simulink model "buck_converter"  (R2020b)
settings: Solver=FixedStepDiscrete  StartTime=0.0  StopTime=1  RelTol=1e-3
undefined symbols (not defined in the file): Acid, Lead
libraries: powerlib x15, powerlib_meascontrol x2, electricdrivelib x1
settings Model: SimulationMode=accelerator  Creator=emin3  LastModifiedBy=emin3
settings DebuggingCC: ArithmeticOperatorsInVariantConditions=warning
settings SFSimCC: CustomCodeUndefinedFunction=UseInterfaceOnly

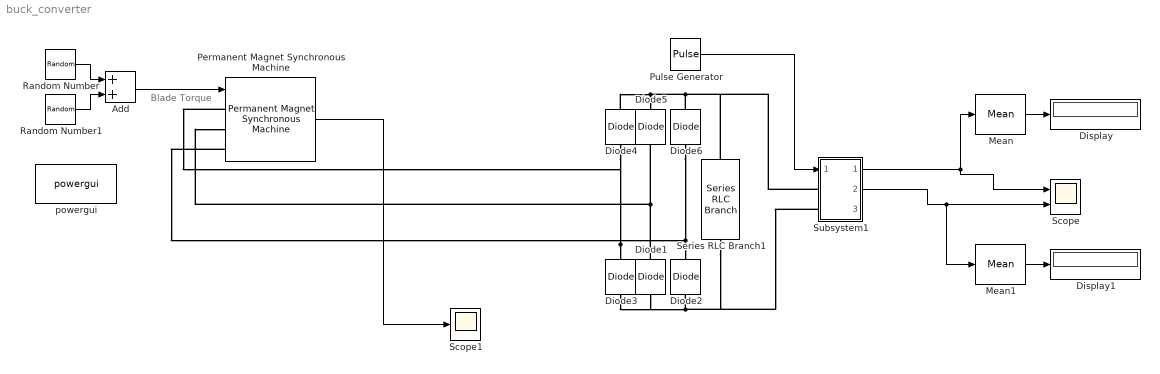
== system buck_converter ==
  note: Blade Torque
  Add : Sum
  Diode{1..6} (6 alike) : powerlib/Power Electronics/Diode  Ron=1e-9  Lon=0  Vf=0.8  IC=0  UseSnubber=0  Rs=1e-6  Cs=250e-9  Measurements=off
  Display : Display
  Display1 : Display
  Mean : powerlib_meascontrol/Measurements/Mean  Freq=60000  Vinit=0  Ts=1e-5
  Mean1 : powerlib_meascontrol/Measurements/Mean  Freq=60000  Vinit=0  Ts=1e-5
  Permanent Magnet Synchronous Machine : powerlib/Machines/Permanent Magnet Synchronous Machine  NbPhases=3  FluxDistribution=Sinusoidal  RotorType=Round  MechanicalLoad=Torque Tm  PresetModel=No  ShowDetailedParameters=on  MeasurementBus=off  Resistance=10.58  Inductance=8.5e-3  dqInductances=[8.5e-3,8.5e-3]  La=0.0167  MachineConstant=Voltage Constant (V_peak L-L / krpm)  Flux=0.60646  VoltageCst=110  TorqueCst=0.90969  Flat=120  Mechanical=[0.00027 0.005024 1 0]  PolePairs=4  InitialConditions=[300,0, 0,0]  InitialConditions5ph=[0 0 0 0 0 0]  RefAngle=90 degrees behind phase A axis (modified Park)  IterativeDiscreteModel=Trapezoidal non iterative  TsBlock=-1  TsPowergui=0
  Pulse Generator : DiscretePulseGenerator  PulseType=Time based  Period=1/6000  PulseWidth=50
  Random Number : RandomNumber  Mean=-1.6  Variance=0.05  SampleTime=1
  Random Number1 : RandomNumber  Variance=0.1  SampleTime=1e-3
  Scope : Scope  NumInputPorts=2
  Scope1 : Scope
  Series RLC Branch1 : powerlib/Elements/Series RLC Branch  LConnTagsString=__new0  RConnTagsString=__new0  BranchType=C  Resistance=20  Inductance=1e-3  SetiL0=off  InitialCurrent=0  Capacitance=1e-6  Setx0=off  InitialVoltage=0  Measurements=None
  Subsystem1 : Subsystem
  powergui : powerlib/powergui  Priority=1  SimulationMode=Discrete  SampleTime=1e-5  frequency=60  Iterations=50  frequencyindice=0  Pbase=100e6  ErrMax=1e-4  UnitsV=kV  UnitsW=MW  buscounter=0  FunctionMessages=off  echomessages=off  EnableUseOfTLC=off  CurrentSourceSwitches=off  DisableSnubberDevices=off  DisableRonSwitches=off  DisableVfSwitches=off  DisplayEquations=off  AutomaticDiscreteSolvers=off  SolverType=Tustin/Backward Euler (TBE)  Interpol=off  ExternalGateDelay=off  methode=off  Ts=100  x0status=blocks  SPID=on  SwTol=0  HookPort=off  NonlinearTolerance=1e-4  nMaxIteration=100  ContinueOnMaxIteration=off  RestoreLinks=warning  ResistiveCurrentMeasurement=off  Frange=[0:2:500]  Ylog=off  Xlog=on  ShowGrid=off  save=off  variable=ZData  structure=0  ZoomFFT=off  StartTime=0.0  cycles=1  DisplayStyle=1  fundamental=60  FreqAxis=off  MaxFrequency=1000  frequencyindicesteady=1  RmsSteady=1  display=off
  wires:
  Random Number/1 -> Add/1
  Add/1 -> Permanent Magnet Synchronous Machine/1
  Random Number1/1 -> Add/2
  Subsystem1/1(Out1) -> Scope/1, Mean/1
  Pulse Generator/1 -> Subsystem1/1(In1)
  Mean/1 -> Display/1
  Mean1/1 -> Display1/1
  Subsystem1/2(Out2) -> Mean1/1, Scope/2
  Permanent Magnet Synchronous Machine/1 -> Scope1/1
  connections:
  Diode6/LConn1 -- Permanent Magnet Synchronous Machine/LConn3 -- Diode2/RConn1
  Diode2/LConn1 -- Diode3/LConn1 -- Diode1/LConn1 -- Subsystem1/LConn2 -- Series RLC Branch1/RConn1
  Diode5/RConn1 -- Diode4/RConn1 -- Subsystem1/LConn1 -- Series RLC Branch1/LConn1 -- Diode6/RConn1
  Diode3/RConn1 -- Permanent Magnet Synchronous Machine/LConn1 -- Diode4/LConn1
  Diode1/RConn1 -- Permanent Magnet Synchronous Machine/LConn2 -- Diode5/LConn1

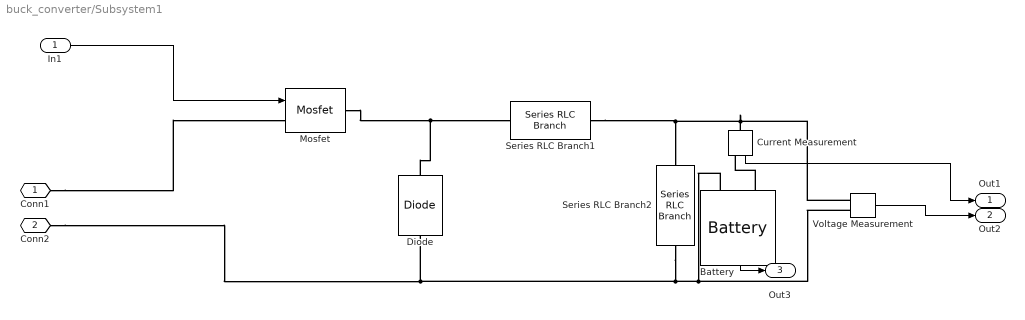
== system buck_converter/Subsystem1 ==
  In1 : Inport
  Battery : electricdrivelib/Extra Sources/Battery  BatType=Lead-Acid  ShowTempParam=off  ThermalPreset=no  ShowAgeParam=off  NomV=24  NomQ=5.4  SOC=50  Batt_Tr=30  PresetModel=on  MaxQ=5.625  MinV=18  FullV=26.1316  Dis_rate=1.08  R=0.044444  Normal_OP=1.6755  expZone="[24.4342        0.018]"  current=[6.5 13 32.5]  Units=Time  Tci=20  NomT=20  T2=-30  MaxQ2=4.8  FullV2=7.1  Normal_OP2=5.655  expZone2="[6.58           1]"  Rca=0.6  ti=2000  Dp=0  Neq0=0  Tsim=1e6  Ta1=25  Qeol=5.4*0.9  Reol=0.013333*1.2  Char_age=[2.3478, 3]  Dis_age=[2.3478, 10]  N1=1500  N2=10500  N3=1000  N4=1400  Ta2=45  N5=950
  Current Measurement : powerlib/Measurements/Current Measurement  PhasorSimulation=off  OutputType=Complex  PSBequivalent=0
  Diode : powerlib/Power Electronics/Diode  Ron=0.001  Lon=0  Vf=0.8  IC=0  UseSnubber=0  Rs=500  Cs=250e-9  Measurements=off
  Mosfet : powerlib/Power Electronics/Mosfet  Ron=0.1  Lon=0  Rd=0.01  Vfd=0  IC=0  Rs=1e5  Cs=inf  Measurements=off
  Series RLC Branch1 : powerlib/Elements/Series RLC Branch  LConnTagsString=__new0  RConnTagsString=__new0  BranchType=L  Resistance=1  Inductance=1e-1  SetiL0=off  InitialCurrent=0  Capacitance=1e-6  Setx0=off  InitialVoltage=0  Measurements=None
  Series RLC Branch2 : powerlib/Elements/Series RLC Branch  LConnTagsString=__new0  RConnTagsString=__new0  BranchType=C  Resistance=1  Inductance=1e-3  SetiL0=off  InitialCurrent=0  Capacitance=1e-6  Setx0=off  InitialVoltage=0  Measurements=None
  Voltage Measurement : powerlib/Measurements/Voltage Measurement  PhasorSimulation=off  OutputType=Complex  PSBequivalent=0
  Conn1 : PMIOPort  Side=Left
  Conn2 : PMIOPort  Port=2  Side=Left
  Out1 : Outport  VectorParamsAs1DForOutWhenUnconnected=off
  Out2 : Outport  Port=2  VectorParamsAs1DForOutWhenUnconnected=off
  Out3 : Outport  Port=3  VectorParamsAs1DForOutWhenUnconnected=off
  wires:
  Current Measurement/1 -> Out1/1
  Voltage Measurement/1 -> Out2/1
  Battery/1 -> Out3/1
  In1/1 -> Mosfet/1
  connections:
  Mosfet/RConn1 -- Diode/RConn1 -- Series RLC Branch1/LConn1
  Battery/LConn1 -- Current Measurement/RConn1
  Battery/LConn2 -- Voltage Measurement/LConn2 -- Series RLC Branch2/RConn1 -- Diode/LConn1 -- Conn2/RConn1
  Voltage Measurement/LConn1 -- Series RLC Branch1/RConn1 -- Series RLC Branch2/LConn1 -- Current Measurement/LConn1
  Conn1/RConn1 -- Mosfet/LConn1
